simulink model "mtq_lib_test"  (R2018b)
settings: Solver=VariableStepAuto  StartTime=0.0  StopTime=10.0  RelTol=1e-3
undefined symbols (not defined in the file or in its folder): simParams
libraries: mtq_lib x1
settings Model: Creator=taylorreynolds  LastModifiedBy=taylorreynolds

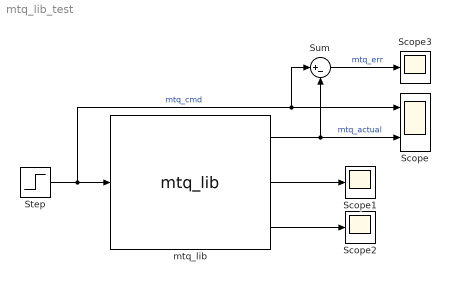
== system mtq_lib_test ==
  Scope : Scope  NumInputPorts=2
  Scope1 : Scope
  Scope2 : Scope
  Scope3 : Scope
  Step : Step  Time=5  Before=[0;0;0]  After=0.5*simParams.actuators.mtq.max_dipoles_Am2  SampleTime=0
  Sum : Sum  Inputs=|+-
  mtq_lib : mtq_lib/mtq_lib  SystemSampleTime=-1
  wires:
  Step/1 -> Sum/1, Scope/1, mtq_lib/1  "mtq_cmd"
  mtq_lib/1 -> Scope/2, Sum/2  "mtq_actual"
  mtq_lib/2 -> Scope1/1
  mtq_lib/3 -> Scope2/1
  Sum/1 -> Scope3/1  "mtq_err"
